simulink library "ccs"  (Simulink 8.1)
settings: Solver=ode1  StartTime=0.0  StopTime=Inf  FixedStep=0.001  RelTol=1e-3
PostLoadFcn:
  | , if any(exist('dsrtsu_mdlpostloadfcn', 'file') == [2, 3, 6]), try dsrtsu_mdlpostloadfcn('Execute', bdroot); catch fprintf('Error in PostLoadFcn (dsrtsu_mdlpostloadfcn) for model "%s":\n %s\n', bdroot, lasterr); end, end,
undefined symbols (not defined in the file or in its folder): C_TICK_TIME_S, ENUM_ACCSTATE_DISABLED, ENUM_ACCSTATE_OFF, ENUM_ACCSTATE_SPEED, ENUM_ACCSTATE_STANDBY, FALSE, KJUD_ACCDeactVehSpeed_kph, KJUD_ACCLargeSpeedDec_kph, KJUD_ACCLargeSpeedInc_kph, KJUD_ACCMaxActSpeed_kph, KJUD_ACCMinActSpeed_kph, KJUD_ACCSpdModifTimer_ms, KJUD_ACCSpeedDec_kph, KJUD_ACCSpeedInc_kph, TRUE, ZERO_FLOAT, ZERO_INT
libraries: hcu_lib x2, simulink x1
settings Model: DSRTSU_INTERNAL_RTI_VER=450  DSRTSU_INTERNAL_RTI_TYPE=rti1401  RTICANMMDATA=struct('GeneralSetupData',struct('modelroot','D:\Projects\ELN150201\Repositories\Taiwan\trunk\AdasDragon\software\sw_development\arch\app\jud','generalsettings',struct('filesettings',struct('destfolder',struct('Name','RTICANMM_FILES','Check',1),'buildfolder',struct('Name','.','Check',1),'AbsDestfolder',struct('Name','D:\Projects\ELN150201\Repositories\Taiwan\trunk\AdasDragon\software\sw_development\arch\app\jud\RTICANMM_FILES'),'AbsBuildfolder',struct('Name','D:\Projects\ELN150201\Repositories\Taiwan\trunk\AdasDragon\software\sw_development\arch\app\jud'))),'options',struct('addpaths',1,'rmpaths',1,'addtrcexclusion',logical(1),'cannavigator',struct('checkmonitoring',0),'show_usrtrc',0,'use_usrtrc',0),'advanced',struct('options',[1 1 1 1 1 1 1 1 1 1 1 1 1 1 1 1 1 1 1 1 1 1 1 1 1 1 1 1 1 1 1 1 1 1 1 1 1 1 1 1 1 1 1 1 1 1 1 1 1 1 1 1 1 1 1 1 1 1 1 1 1 1 1 1 1 1 1 1 1 1 1 1 1 1 1 1 1 1 1 1 1 1 1 1 1 1 1 1 1 1 1 1 1 1 1 1 1 1 1 1]),'MPSetup',{{}},'modelname','ccs','block','ccs'))  DSRTSU_INTERNAL_RTIFPGA=40  Creator=AT015411  LastModifiedBy=AT015086

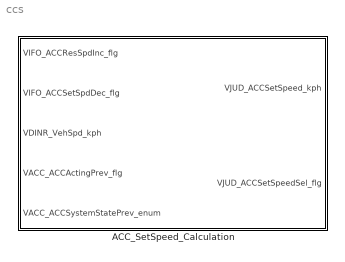
== system ccs ==
  ACC_SetSpeed_Calculation : Subsystem

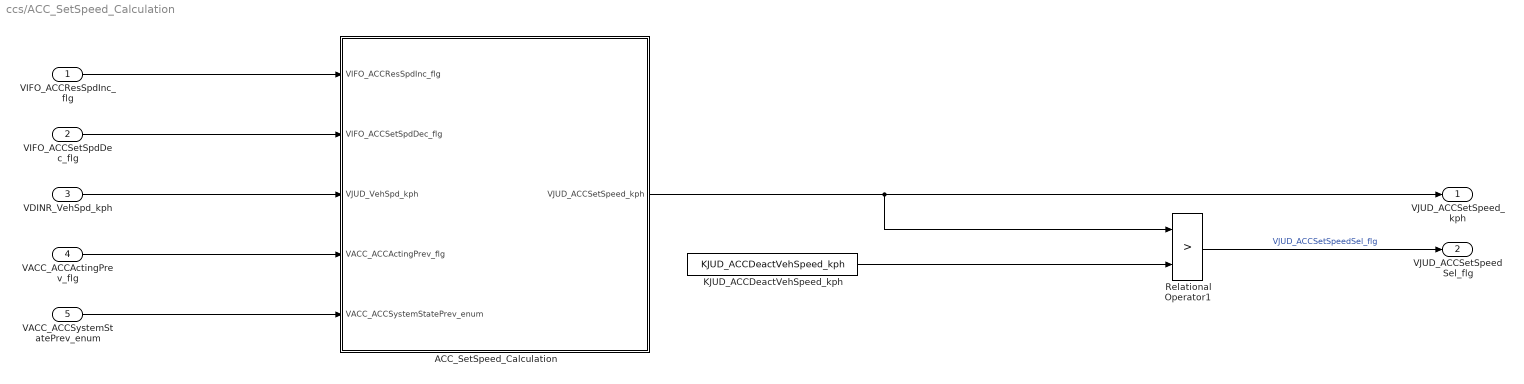
== system ccs/ACC_SetSpeed_Calculation ==
  VIFO_ACCResSpdInc_flg : Inport
  VIFO_ACCSetSpdDec_flg : Inport  Port=2
  VDINR_VehSpd_kph : Inport  Port=3
  VACC_ACCActingPrev_flg : Inport  Port=4
  VACC_ACCSystemStatePrev_enum : Inport  Port=5
  ACC_SetSpeed_Calculation : Subsystem
  KJUD_ACCDeactVehSpeed_kph : Constant  Value=KJUD_ACCDeactVehSpeed_kph
  Relational Operator1 : RelationalOperator  Operator=>  OutDataTypeStr=boolean
  VJUD_ACCSetSpeed_kph : Outport
  VJUD_ACCSetSpeedSel_flg : Outport  Port=2
  wires:
  VACC_ACCActingPrev_flg/1 -> ACC_SetSpeed_Calculation/4(VACC_ACCActingPrev_flg)
  VACC_ACCSystemStatePrev_enum/1 -> ACC_SetSpeed_Calculation/5(VACC_ACCSystemStatePrev_enum)
  ACC_SetSpeed_Calculation/1(VJUD_ACCSetSpeed_kph) -> VJUD_ACCSetSpeed_kph/1, Relational Operator1/1
  KJUD_ACCDeactVehSpeed_kph/1 -> Relational Operator1/2
  Relational Operator1/1 -> VJUD_ACCSetSpeedSel_flg/1  "VJUD_ACCSetSpeedSel_flg"
  VIFO_ACCSetSpdDec_flg/1 -> ACC_SetSpeed_Calculation/2(VIFO_ACCSetSpdDec_flg)
  VIFO_ACCResSpdInc_flg/1 -> ACC_SetSpeed_Calculation/1(VIFO_ACCResSpdInc_flg)
  VDINR_VehSpd_kph/1 -> ACC_SetSpeed_Calculation/3(VJUD_VehSpd_kph)

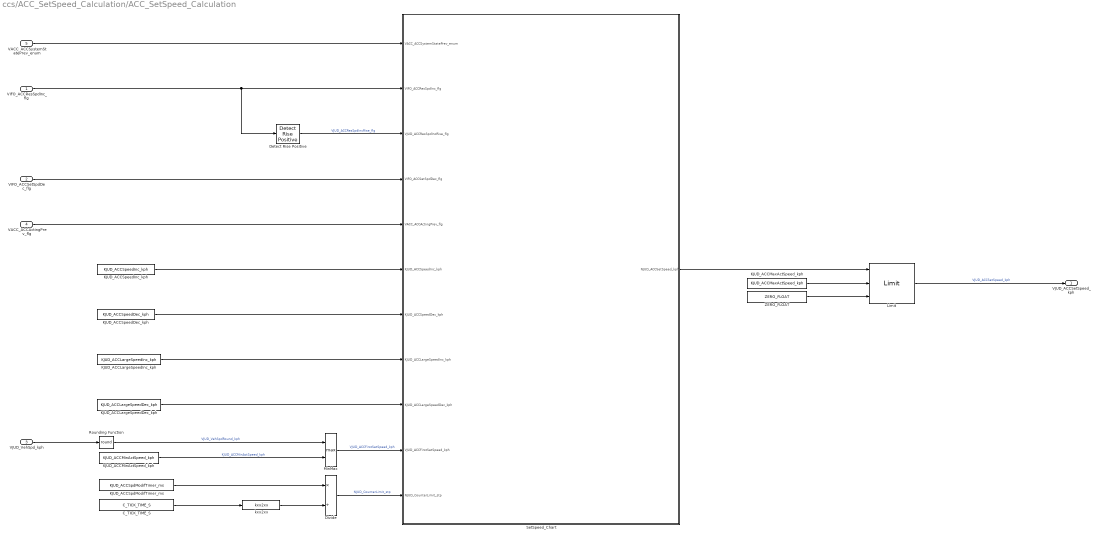
== system ccs/ACC_SetSpeed_Calculation/ACC_SetSpeed_Calculation ==
  VIFO_ACCResSpdInc_flg : Inport
  VIFO_ACCSetSpdDec_flg : Inport  Port=2
  VJUD_VehSpd_kph : Inport  Port=3
  VACC_ACCActingPrev_flg : Inport  Port=4
  VACC_ACCSystemStatePrev_enum : Inport  Port=5
  C_TICK_TIME_S : Constant  Value=C_TICK_TIME_S  OutDataTypeStr=single
  Detect Rise Positive : simulink/Logic and Bit Operations/Detect Rise Positive  vinit=0  InputProcessing=Inherited  OutDataTypeStr=boolean
  Divide : Product  Inputs=*/
  KJUD_ACCLargeSpeedDec_kph : Constant  Value=KJUD_ACCLargeSpeedDec_kph
  KJUD_ACCLargeSpeedInc_kph : Constant  Value=KJUD_ACCLargeSpeedInc_kph
  KJUD_ACCMaxActSpeed_kph : Constant  Value=KJUD_ACCMaxActSpeed_kph
  KJUD_ACCMinActSpeed_kph : Constant  Value=KJUD_ACCMinActSpeed_kph
  KJUD_ACCSpdModifTimer_ms : Constant  Value=KJUD_ACCSpdModifTimer_ms  OutDataTypeStr=single
  KJUD_ACCSpeedDec_kph : Constant  Value=KJUD_ACCSpeedDec_kph
  KJUD_ACCSpeedInc_kph : Constant  Value=KJUD_ACCSpeedInc_kph
  Limit : hcu_lib/Limit  SystemSampleTime=-1
  MinMax : MinMax  Function=max  Inputs=2
  Rounding Function : Rounding  Operator=round
  SetSpeed_Chart : Stateflow chart  TreatAsAtomicUnit=on
  ZERO_FLOAT : Constant  Value=ZERO_FLOAT
  kxx2xx : hcu_lib/kxx2xx
  VJUD_ACCSetSpeed_kph : Outport  OutputWhenDisabled=reset  InitialOutput=0
  wires:
  MinMax/1 -> SetSpeed_Chart/10(VJUD_ACCFirstSetSpeed_kph)  "VJUD_ACCFirstSetSpeed_kph"
  Detect Rise Positive/1 -> SetSpeed_Chart/3(VJUD_ACCResSpdIncRise_flg)  "VJUD_ACCResSpdIncRise_flg"
  VACC_ACCSystemStatePrev_enum/1 -> SetSpeed_Chart/1(VACC_ACCSystemStatePrev_enum)
  KJUD_ACCLargeSpeedDec_kph/1 -> SetSpeed_Chart/9(KJUD_ACCLargeSpeedDec_kph)
  KJUD_ACCLargeSpeedInc_kph/1 -> SetSpeed_Chart/8(KJUD_ACCLargeSpeedInc_kph)
  VIFO_ACCResSpdInc_flg/1 -> Detect Rise Positive/1, SetSpeed_Chart/2(VIFO_ACCResSpdInc_flg)
  VIFO_ACCSetSpdDec_flg/1 -> SetSpeed_Chart/4(VIFO_ACCSetSpdDec_flg)
  Limit/1 -> VJUD_ACCSetSpeed_kph/1  "VJUD_ACCSetSpeed_kph"
  SetSpeed_Chart/1(NJUD_ACCSetSpeed_kph) -> Limit/1
  ZERO_FLOAT/1 -> Limit/3
  KJUD_ACCMaxActSpeed_kph/1 -> Limit/2
  Divide/1 -> SetSpeed_Chart/11(NJUD_CounterLimit_stp)  "NJUD_CounterLimit_stp"
  kxx2xx/1 -> Divide/2
  C_TICK_TIME_S/1 -> kxx2xx/1
  KJUD_ACCSpdModifTimer_ms/1 -> Divide/1
  VACC_ACCActingPrev_flg/1 -> SetSpeed_Chart/5(VACC_ACCActingPrev_flg)
  Rounding Function/1 -> MinMax/1  "VJUD_VehSpdRound_kph"
  KJUD_ACCMinActSpeed_kph/1 -> MinMax/2  "KJUD_ACCMinActSpeed_kph"
  VJUD_VehSpd_kph/1 -> Rounding Function/1
  KJUD_ACCSpeedInc_kph/1 -> SetSpeed_Chart/6(KJUD_ACCSpeedInc_kph)
  KJUD_ACCSpeedDec_kph/1 -> SetSpeed_Chart/7(KJUD_ACCSpeedDec_kph)

== stateflow chart ACC_SetSpeed_Calculation/ACC_SetSpeed_Calculation/SetSpeed_Chart ==
  state INITIALIZATION
    en:
    NJUD_ACCSetSpeed_kph = ZERO_FLOAT;
  state SPEED_MODIF
    state INC_SPEED
      en:
      NJUD_LargeSpeedInc_flg=FALSE;
      NJUD_ACCSetSpeed_kph = NJUD_ACCSetSpeed_kph + KJUD_ACCSpeedInc_kph;
      ex:
      NJUD_LargeSpeedInc_flg=FALSE;
      state INC_LARGE_STEP
        en:
        NJUD_ACCSetSpeed_kph = NJUD_ACCSetSpeed_kph + KJUD_ACCLargeSpeedInc_kph;
      state INC_COUNT
        en:
        NJUD_IncCountLocal_stp = ZERO_INT;
        du:
        NJUD_IncCountLocal_stp = NJUD_IncCountLocal_stp + 1;
      state INC_FIRST_STEP
        en:
        NJUD_ACCSetSpeed_kph = NJUD_ACCSetSpeed_kph + KJUD_ACCLargeSpeedInc_kph -KJUD_ACCSpeedInc_kph;
        NJUD_LargeSpeedInc_flg=TRUE;
      (default) -> INC_COUNT
      INC_COUNT -> INC_FIRST_STEP [order 2] : [NJUD_IncCountLocal_stp > NJUD_CounterLimit_stp ...
          | && NJUD_LargeSpeedInc_flg == FALSE]
      INC_FIRST_STEP -> INC_COUNT
      INC_COUNT -> INC_LARGE_STEP [order 1] : [NJUD_IncCountLocal_stp > NJUD_CounterLimit_stp ...
          | && NJUD_LargeSpeedInc_flg == TRUE]
      INC_LARGE_STEP -> INC_COUNT
    state DEC_SPEED
      en:
      NJUD_LargeSpeedDec_flg=FALSE;
      NJUD_ACCSetSpeed_kph = NJUD_ACCSetSpeed_kph - KJUD_ACCSpeedDec_kph;
      ex:
      NJUD_LargeSpeedDec_flg=FALSE;
      state DEC_LARGE_STEP
        en:
        NJUD_ACCSetSpeed_kph = NJUD_ACCSetSpeed_kph - KJUD_ACCLargeSpeedDec_kph;
      state DEC_COUNT
        en:
        NJUD_DecCountLocal_stp = ZERO_INT;
        du:
        NJUD_DecCountLocal_stp = NJUD_DecCountLocal_stp + 1;
      state DEC_FIRST_STEP
        en:
        NJUD_ACCSetSpeed_kph = NJUD_ACCSetSpeed_kph - KJUD_ACCLargeSpeedDec_kph +KJUD_ACCSpeedDec_kph;
        NJUD_LargeSpeedDec_flg=TRUE;
      (default) -> DEC_COUNT
      DEC_COUNT -> DEC_FIRST_STEP [order 2] : [NJUD_DecCountLocal_stp > NJUD_CounterLimit_stp ...
          | && NJUD_LargeSpeedDec_flg == FALSE]
      DEC_FIRST_STEP -> DEC_COUNT
      DEC_COUNT -> DEC_LARGE_STEP [order 1] : [NJUD_DecCountLocal_stp > NJUD_CounterLimit_stp ...
          | && NJUD_LargeSpeedDec_flg == TRUE]
      DEC_LARGE_STEP -> DEC_COUNT
    state HOLD
    (default) -> HOLD
    HOLD -> INC_SPEED [order 1] : [VJUD_ACCResSpdIncRise_flg == TRUE...
        | && VACC_ACCSystemStatePrev_enum == ENUM_ACCSTATE_SPEED]
    INC_SPEED -> HOLD : [VIFO_ACCResSpdInc_flg==FALSE]
    HOLD -> DEC_SPEED [order 2] : [VIFO_ACCSetSpdDec_flg == TRUE...
        | && VACC_ACCSystemStatePrev_enum == ENUM_ACCSTATE_SPEED]
    DEC_SPEED -> HOLD : [VIFO_ACCSetSpdDec_flg==FALSE]
  state SET_SPEED
    en:
    NJUD_ACCSetSpeed_kph = VJUD_ACCFirstSetSpeed_kph;
  (default) -> INITIALIZATION
  INITIALIZATION -> SET_SPEED : [VACC_ACCSystemStatePrev_enum == ENUM_ACCSTATE_STANDBY...
      | && VIFO_ACCSetSpdDec_flg == TRUE ]
  SET_SPEED -> SPEED_MODIF [order 2] : [VACC_ACCActingPrev_flg == TRUE]
  SET_SPEED -> INITIALIZATION [order 1] : [VACC_ACCSystemStatePrev_enum == ENUM_ACCSTATE_OFF...
      | || VACC_ACCSystemStatePrev_enum == ENUM_ACCSTATE_DISABLED]
  HOLD -> SET_SPEED [order 3] : [VIFO_ACCSetSpdDec_flg==TRUE]
  SPEED_MODIF -> INITIALIZATION : [VACC_ACCSystemStatePrev_enum == ENUM_ACCSTATE_OFF...
      | || VACC_ACCSystemStatePrev_enum == ENUM_ACCSTATE_DISABLED]
  data: VACC_ACCSystemStatePrev_enum input double; VIFO_ACCResSpdInc_flg input double; VJUD_ACCResSpdIncRise_flg input double; VIFO_ACCSetSpdDec_flg input double; NJUD_ACCSetSpeed_kph output single =0; VACC_ACCActingPrev_flg input boolean; KJUD_ACCSpeedInc_kph input single; KJUD_ACCSpeedDec_kph input single; KJUD_ACCLargeSpeedInc_kph input double; KJUD_ACCLargeSpeedDec_kph input double; VJUD_ACCFirstSetSpeed_kph input double; NJUD_CounterLimit_stp input single; ZERO_FLOAT parameter single; TRUE parameter boolean; ZERO_INT parameter double; FALSE parameter boolean; NJUD_LargeSpeedDec_flg local boolean; NJUD_DecCountLocal_stp local single; NJUD_LargeSpeedInc_flg local boolean; NJUD_IncCountLocal_stp local single; ENUM_ACCSTATE_STANDBY parameter uint8; ENUM_ACCSTATE_SPEED parameter uint8; ENUM_ACCSTATE_OFF parameter uint8; ENUM_ACCSTATE_DISABLED parameter uint8
